simulink library "SendToPDB"  (R2016b)
settings: Solver=VariableStepAuto  StartTime=0.0  StopTime=10.0  RelTol=1e-3
settings Model: Creator=Nathan  LastModifiedBy=march

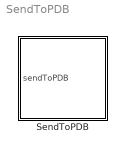
== system SendToPDB ==
  SendToPDB : Subsystem

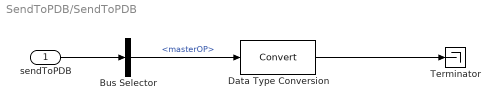
== system SendToPDB/SendToPDB ==
  sendToPDB : Inport  OutDataTypeStr=Bus: EtherCATSendToPDB  BusOutputAsStruct=on
  Bus Selector : BusSelector  OutputSignals=masterOP
  Data Type Conversion : DataTypeConversion
  Terminator : Terminator
  wires:
  Data Type Conversion/1 -> Terminator/1
  Bus Selector/1 -> Data Type Conversion/1  "<masterOP>"
  sendToPDB/1 -> Bus Selector/1
